simulink model "motore"  (R2019b)
settings: Solver=VariableStepAuto  StartTime=0.0  StopTime=10.0  RelTol=1e-3
model mask{C_Q_coeff=7}
model workspace (MAT data in the model file):
  C_Q_coeff = 0
  Var = 3
undefined symbols (not defined in the file or in its folder): omega, thrust, torque
settings Model: ParameterArgumentNames=C_Q_coeff  OrderedModelArguments=off  Creator=Alessandro  LastModifiedBy=Alessandro

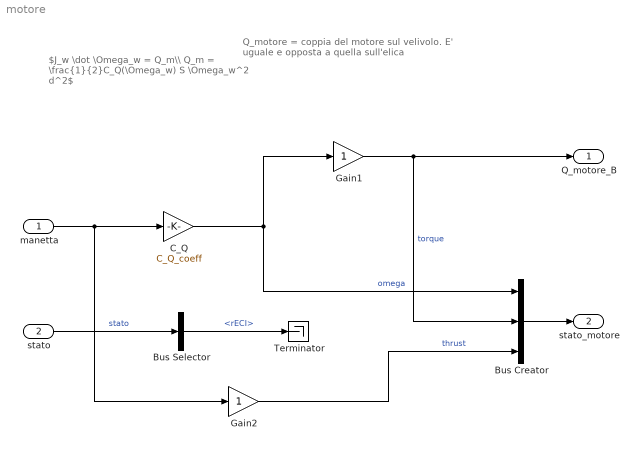
== system motore ==
  note: Q_motore = coppia del motore sul velivolo.
      | E' uguale e opposta a quella sull'elica
  note: $J_w \dot \Omega_w = Q_m\\ Q_m = \frac{1}{2}C_Q(\Omega_w) S \Omega_w^2 d^2$
  manetta : Inport  PortDimensions=1
  stato : Inport  Port=2  OutDataTypeStr=Bus: stato6DoF  PortDimensions=1  LockScale=on  BusOutputAsStruct=on
  Bus Creator : BusCreator  Inputs=omega,torque,thrust  OutDataTypeStr=Bus: BUS_statoMotore
  Bus Selector : BusSelector  OutputSignals=rECI
  C_Q : Gain  Gain=C_Q_coeff  ParamMin=-1000  ParamMax=1000  ParamDataTypeStr=double
  Gain1 : Gain
  Gain2 : Gain
  Terminator : Terminator
  Q_motore_B : Outport  OutDataTypeStr=double  Unit=N*m  PortDimensions=1
  stato_motore : Outport  Port=2  OutDataTypeStr=Bus: BUS_statoMotore  Unit=N*m  PortDimensions=1  LockScale=on  BusOutputAsStruct=on
  wires:
  stato/1 -> Bus Selector/1  "stato"
  manetta/1 -> Gain2/1, C_Q/1
  Gain1/1 -> Bus Creator/2, Q_motore_B/1  "torque"
  Bus Selector/1 -> Terminator/1  "<rECI>"
  Bus Creator/1 -> stato_motore/1
  C_Q/1 -> Gain1/1, Bus Creator/1  "omega"
  Gain2/1 -> Bus Creator/3  "thrust"
